simulink model "third"  (R2020b)
settings: Solver=VariableStepAuto  StartTime=0.0  StopTime=10.0  RelTol=1e-3
undefined symbols (not defined in the file): a, b
settings Model: Creator=priyaD  LastModifiedBy=priyaD

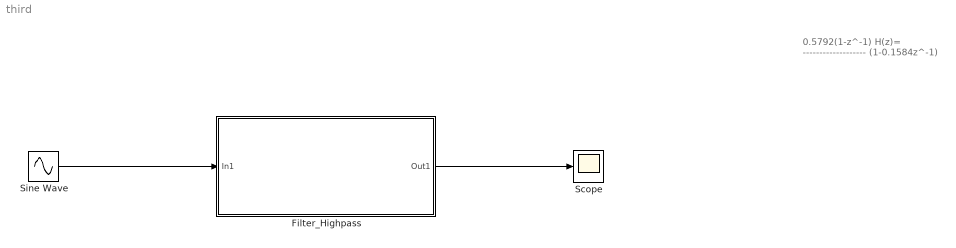
== system third ==
  note: 0.5792(1-z^-1)
      | H(z)= -------------------
      | (1-0.1584z^-1)
  Filter_Highpass : Subsystem
  Scope : Scope
  Sine Wave : Sin  SampleTime=0
  wires:
  Sine Wave/1 -> Filter_Highpass/1(In1)
  Filter_Highpass/1(Out1) -> Scope/1

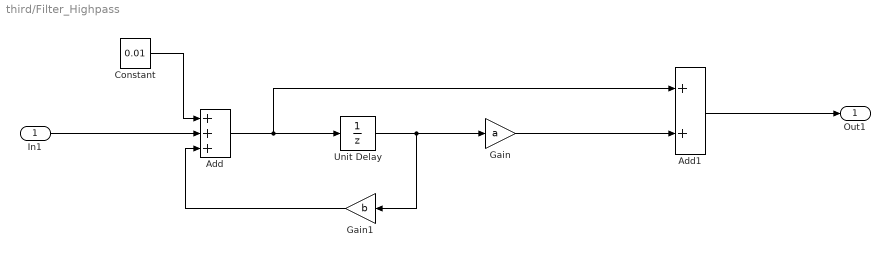
== system third/Filter_Highpass ==
  In1 : Inport
  Add : Sum  Inputs=+++
  Add1 : Sum
  Constant : Constant  Value=0.01
  Gain : Gain  Gain=a
  Gain1 : Gain  Gain=b
  Unit Delay : UnitDelay  SampleTime=-1  HasFrameUpgradeWarning=on
  Out1 : Outport
  wires:
  Unit Delay/1 -> Gain1/1, Gain/1
  Add/1 -> Add1/1, Unit Delay/1
  Gain1/1 -> Add/3
  Constant/1 -> Add/1
  In1/1 -> Add/2
  Gain/1 -> Add1/2
  Add1/1 -> Out1/1
